simulink model "direct_torque_control"  (Simulink 8.0)
settings: Solver=ode45  StartTime=0.0  StopTime=.4  MaxStep=6e-7  RelTol=1e-3
InitFcn:
  | clear;
  | warning off;
  | wmo=0.0;       %initial speed
  | fso=.996;        %initial stator flux
  | Vdc=700;
  | wo=2*pi*50;
  | 
  | %switching table for DTC
  | a(:,:,1) =[4 0 2;5 7 3];
  | a(:,:,2) =[5 7 6;1 0 2];
  | a(:,:,3) =[1 0 4;3 7 6];
  | a(:,:,4) =[3 7 5;2 0 4];
  | a(:,:,5) =[2 0 1;6 7 5];
  | a(:,:,6) =[6 7 3;4 0 1];
  | clc;
  | %
StopFcn:
  | close all;
  | scrsz = get(0,'ScreenSize');
  | 
  | figure('Name',' Results','OuterPosition',[1 100 scrsz(3)*0.75 scrsz(4)*0.75]);
  | 
  | subplot(1,2,1);
  | plot(fs(:,1),fs(:,2),'-r',fr(:,1),fr(:,2),'-b');
  | axis equal;
  | grid on;
  | title('Flux Spave Vector Trajectory');
  | text(.8,-.85,'rotor flux','color','b');
  | text(-1,-.85,'stator flux','color','r');
  | %figure(2);
  | subplot(1,2,2);
  | plot(an(:,1),unwrap(an(:,2)),'r');
  | grid on;
  | xlabel('Time [s]');
  | ylabel('Rotor flux angle [rad]');
undefined symbols (not defined in the file): a
libraries: simulink x1
settings Model: Creator=Syed Abdul Rahman Kashif  LastModifiedBy=AbdulRahman
settings DataIOCC: SignalLoggingSaveFormat=ModelDataLogs  SignalLoggingName=sigsOut
settings OptimizationCC: BlockReduction=off  BooleanDataType=off
settings DebuggingCC: SaveWithParameterizedLinksMsg=none  SignalResolutionControl=TryResolveAllWithWarning  SolverPrmCheckMsg=none  MultiTaskDSMMsg=warning  MultiTaskCondExecSysMsg=none  FcnCallInpInsideContextMsg=UseLocalSettings  StrictBusMsg=None
settings HardwareCC: TargetUnknown=on
settings RTWCC: IncludeERTFirstTime=on
settings GRTTargetCC: CombineOutputUpdateFcns=off  GRTInterface=on

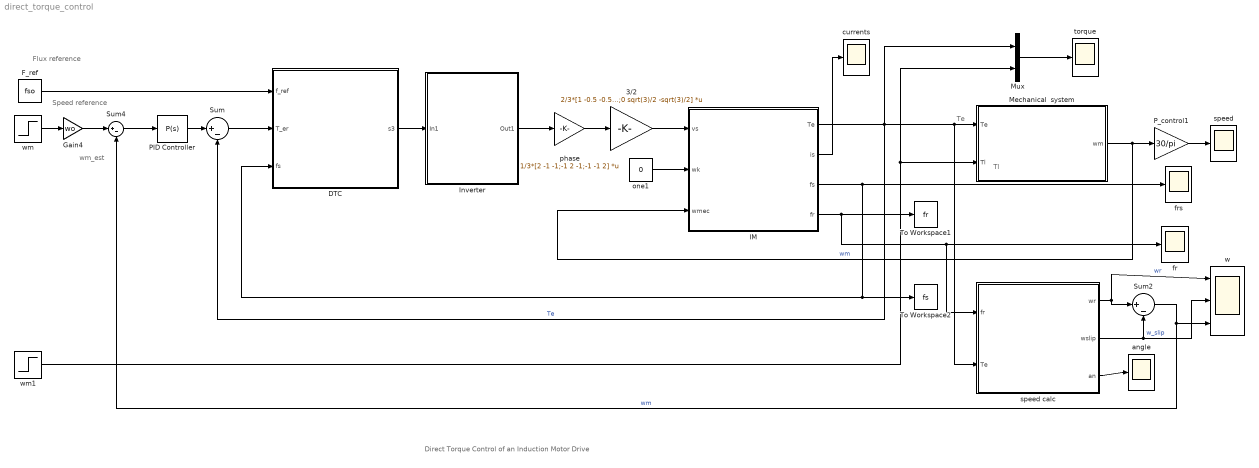
== system direct_torque_control ==
  note: Direct Torque Control of an Induction Motor Drive
  note: Flux reference
  note: Speed reference
  note: Te
  note: Tl
  note: wm_est
  3/2 : Gain  Gain=2/3*[1 -0.5 -0.5;0 sqrt(3)/2 -sqrt(3)/2]  Multiplication=Matrix(K*u)  SaturateOnIntegerOverflow=on  OutDataTypeStr=Inherit: Same as input  ParamDataTypeStr=Inherit: Same as input
  DTC : Subsystem
      mask Display: disp('DTC\ncontroller')
  F_ref : Constant  Value=fso
  Gain4 : Gain  Gain=wo  SaturateOnIntegerOverflow=on  OutDataTypeStr=Inherit: Same as input  ParamDataTypeStr=Inherit: Same as input
  IM : Subsystem  mask{Rs=1.77, Rr=1.34, Lsl=13.93e-3, Lrl=12.12e-3, Lm=369e-3, p=4}
      mask prompts: Rs "Stator resistance [Ohm]"; Rr "Rotor resistance [Ohm]"; Lsl "Stator leakage inductance [H]"; Lrl "Rotor leakage inductance [H]"; Lm "Magnetizing inductance [H]"; p "Number of poles"
      mask Display: disp('INDUCTION\nMOTOR')
  Inverter : Subsystem
  Mechanical  system : Subsystem  mask{J=0.025, Bm=1e-5}
      mask prompts: J "Moment of inertia [Kg.m^2]"; Bm "Torque-speed coefficient"
      mask Display: disp('MECHANICAL\nSYSTEM')
  Mux : Mux  Inputs=2
  PID Controller : simulink/Continuous/PID Controller  Controller=P  TimeDomain=Continuous-time  SampleTime=1  IntegratorMethod=Forward Euler  FilterMethod=Forward Euler  Form=Parallel  P=4  I=1  D=0  N=100  InitialConditionSource=internal  InitialConditionForIntegrator=0  InitialConditionForFilter=0  ExternalReset=none  LimitOutput=on  UpperSaturationLimit=30  LowerSaturationLimit=-30  LinearizeAsGain=on  AntiWindupMode=none  Kb=1  TrackingMode=off  Kt=1  PParamMin=[]  PParamMax=[]  IParamMin=[]  IParamMax=[]  DParamMin=[]  DParamMax=[]  NParamMin=[]  NParamMax=[]  KbParamMin=[]  KbParamMax=[]  KtParamMin=[]  KtParamMax=[]  POutMin=[]  POutMax=[]  IOutMin=[]  IOutMax=[]  DOutMin=[]  DOutMax=[]  NOutMin=[]  NOutMax=[]  KbOutMin=[]  KbOutMax=[]  KtOutMin=[]  KtOutMax=[]  IntegratorOutMin=[]  IntegratorOutMax=[]  FilterOutMin=[]  FilterOutMax=[]  SumOutMin=[]  SumOutMax=[]  SumI1OutMin=[]  SumI1OutMax=[]  SumI2OutMin=[]  SumI2OutMax=[]  SumI3OutMin=[]  SumI3OutMax=[]  SumDOutMin=[]  SumDOutMax=[]  SaturationOutMin=[]  SaturationOutMax=[]  IntegratorContinuousStateAttributes=''  IntegratorStateMustResolveToSignalObject=off  IntegratorRTWStateStorageClass=Auto  FilterContinuousStateAttributes=''  FilterStateMustResolveToSignalObject=off  FilterRTWStateStorageClass=Auto
  P_control1 : Gain  Gain=30/pi  SaturateOnIntegerOverflow=on  OutDataTypeStr=Inherit: Same as input  ParamDataTypeStr=Inherit: Same as input
  Sum : Sum  Inputs=|+-  SaturateOnIntegerOverflow=on
  Sum2 : Sum  Inputs=|+-  SaturateOnIntegerOverflow=on
  Sum4 : Sum  Inputs=|+-  SaturateOnIntegerOverflow=on  InputSameDT=on  OutDataTypeStr=Inherit: Same as first input
  To Workspace1 : ToWorkspace  VariableName=fr  SampleTime=-1
      settings: Decimation=2
  To Workspace2 : ToWorkspace  VariableName=fs  SampleTime=-1
      settings: Decimation=2
  angle : Scope
      settings: TimeRange=0.4  YMin=-3.5  YMax=3.5  SaveName=an  MaxDataPoints=20000  Decimation=20
  currents : Scope
      settings: TimeRange=0.4  YMin=-3.5  YMax=3.5  MaxDataPoints=20000  Decimation=20
  fr : Scope
      settings: TimeRange=1  YMin=-1.5  YMax=1.5  MaxDataPoints=20000  Decimation=20
  frs : Scope
      settings: TimeRange=2  YMin=-1.1  YMax=1.1  SaveName=ScopeData4  MaxDataPoints=20000  Decimation=20
  one1 : Constant  Value=0
  phase : Gain  Gain=1/3*[2 -1 -1;-1 2 -1;-1 -1 2]  Multiplication=Matrix(K*u)  SaturateOnIntegerOverflow=on  OutDataTypeStr=Inherit: Same as input  ParamDataTypeStr=Inherit: Same as input
  speed : Scope
      settings: TimeRange=0.4  YMin=0  YMax=1500  SaveName=ScopeData2  MaxDataPoints=20000  Decimation=20
  speed calc : Subsystem
      mask Display: disp('Speed\nEstimator')
  torque : Scope
      settings: TimeRange=0.4  YMin=-2.5  YMax=32.5  SaveName=ScopeData3  MaxDataPoints=20000  Decimation=20
  w : Scope  NumInputPorts=3
      settings: TimeRange=0.4  YMin=0~-2.5~-50  YMax=350~20~350  SaveName=ScopeData6
  wm : Step  Time=.05  Before=wmo  After=.8  SampleTime=0
  wm1 : Step  Time=.3  After=12  SampleTime=0
  wires:
  F_ref/1 -> DTC/1(f_ref)
  3/2/1 -> IM/1(vs)
  IM/3(fs) -> frs/1, To Workspace2/1, DTC/3(fs)
  one1/1 -> IM/2(wk)
  IM/1(Te) -> Mechanical  system/1(Te), speed calc/2(Te), Sum/2, Mux/1  "Te"
  Mechanical  system/1(wm) -> IM/3(wmec), P_control1/1  "wm"
  IM/2(is) -> currents/1
  wm/1 -> Gain4/1
  Sum/1 -> DTC/2(T_er)
  Mux/1 -> torque/1
  IM/4(fr) -> To Workspace1/1, fr/1, speed calc/1(fr)
  wm1/1 -> Mechanical  system/2(Tl), Mux/2
  speed calc/1(wr) -> Sum2/1, w/1  "wr"
  speed calc/2(wslip) -> w/2, Sum2/2  "w_slip"
  Sum2/1 -> Sum4/2, w/3  "wm"
  phase/1 -> 3/2/1
  Gain4/1 -> Sum4/1
  P_control1/1 -> speed/1
  speed calc/3(an) -> angle/1
  Sum4/1 -> PID Controller/1
  PID Controller/1 -> Sum/1
  DTC/1(s3) -> Inverter/1(In1)
  Inverter/1(Out1) -> phase/1

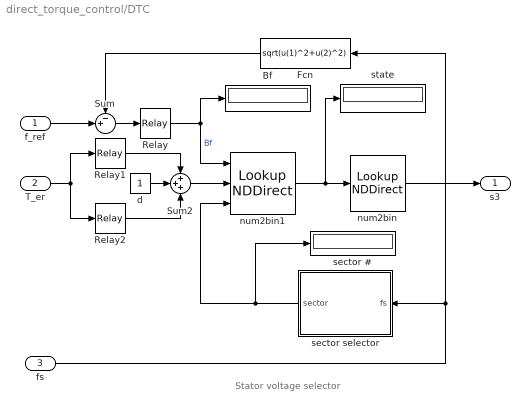
== system direct_torque_control/DTC ==
  note: Stator voltage selector
  f_ref : Inport
  T_er : Inport  Port=2
  fs : Inport  Port=3
  Bf : Display
  Fcn : Fcn  Expr=sqrt(u(1)^2+u(2)^2)
  Relay : Relay  OnSwitchValue=.02  OffSwitchValue=-.02
  Relay1 : Relay  OnSwitchValue=.2  OffSwitchValue=0  ZeroCross=off
  Relay2 : Relay  OnSwitchValue=0  OffSwitchValue=-.2  OnOutputValue=0  OffOutputValue=-1  ZeroCross=off
  Sum : Sum  Inputs=-+|  SaturateOnIntegerOverflow=on  InputSameDT=on  OutDataTypeStr=Inherit: Same as first input
  Sum2 : Sum  Inputs=+++  SaturateOnIntegerOverflow=on  InputSameDT=on  OutDataTypeStr=Inherit: Same as first input
  d : Constant
  num2bin : LookupNDDirect  InputsSelectThisObjectFromTable=Column  Table=[0 0 0;1 0 0;0 1 0;1 1 0;0 0 1;1 0 1;0 1 1;1 1 1]'  DiagnosticForOutOfRangeInput=Error
  num2bin1 : LookupNDDirect  NumberOfTableDimensions=3  Table=a  DiagnosticForOutOfRangeInput=Error
  sector # : Display
  sector selector : Subsystem
  state : Display
  s3 : Outport
  wires:
  num2bin1/1 -> state/1, num2bin/1
  Sum/1 -> Relay/1
  Relay/1 -> Bf/1, num2bin1/1  "Bf"
  Fcn/1 -> Sum/1
  Sum2/1 -> num2bin1/2
  Relay1/1 -> Sum2/1
  Relay2/1 -> Sum2/3
  d/1 -> Sum2/2
  T_er/1 -> Relay2/1, Relay1/1
  f_ref/1 -> Sum/2
  num2bin/1 -> s3/1
  fs/1 -> Fcn/1, sector selector/1(fs)
  sector selector/1(sector) -> num2bin1/3, sector #/1

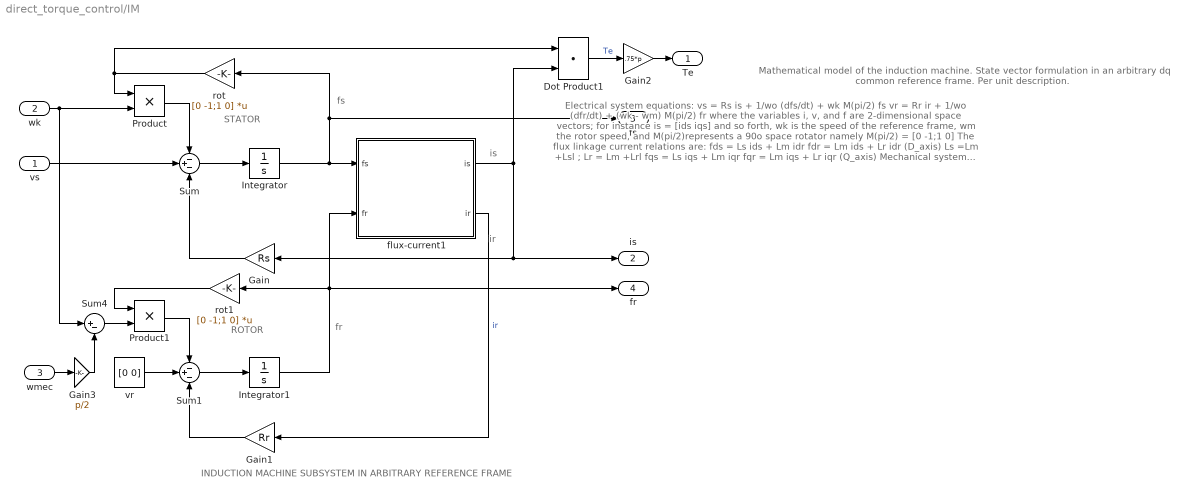
== system direct_torque_control/IM ==
  note: ROTOR
  note: STATOR
  note: fs
  note: fr
  note: is
  note: INDUCTION MACHINE SUBSYSTEM IN ARBITRARY REFERENCE FRAME
  note: ir
  note: Mathematical model of the induction machine.
      | State vector formulation in an arbitrary dq common reference frame.
      | Per unit description.
  note: Electrical  system equations:
      |             vs = Rs is + 1/wo (dfs/dt) + wk M(pi/2) fs
      |             vr  = Rr ir  + 1/wo (dfr/dt)  + (wk - wm) M(pi/2) fr
      |       where the variables i, v, and f are 2-dimensional space vectors; for instance
      |             is = [ids iqs] and so forth,
      |       wk is the speed of the reference frame, wm the rotor speed,
      |       and M(pi/2)represents a 90o space rotator namely M(pi/2) = [0 -1;1 0]
      |
      |     The flux linkage current relations are:
      |           fds = Ls ids + Lm idr
      |           fdr =  Lm ids + Lr idr          (D_axis)
      |                                                                        Ls =Lm +Lsl  ; Lr = Lm +Lrl
      |           fqs = Ls iqs + Lm iqr
      |           fqr  = Lm iqs + Lr iqr         (Q_axis)
      |
      |  Mechanical system equations:
      |              Te = 2H (dwm/dt ) + Bm wm + Tl
      |             where Te = fs (cross) is = M(pi/2) fs (dot) is = fds iqs - fqs ids
      |                               = fs x is = M(pi/2) fs . is
      |                               = ir x fr   = Lm (ir x is) = Lm/Lr (fr x is)
      |                               = 1/Lm' (fr x fs)        Lm' =Lm c/(1-c)   c = 1 - Lm^2/(Ls Lr)
  vs : Inport
  wk : Inport  Port=2
  wmec : Inport  Port=3
  Dot Product1 : DotProduct  InputSameDT=on  OutDataTypeStr=Inherit: Inherit via internal rule
  Gain : Gain  Gain=Rs  SaturateOnIntegerOverflow=on  OutDataTypeStr=Inherit: Same as input  ParamDataTypeStr=Inherit: Same as input
  Gain1 : Gain  Gain=Rr  SaturateOnIntegerOverflow=on  OutDataTypeStr=Inherit: Same as input  ParamDataTypeStr=Inherit: Same as input
  Gain2 : Gain  Gain=.75*p  SaturateOnIntegerOverflow=on  OutDataTypeStr=Inherit: Same as input  ParamDataTypeStr=Inherit: Same as input
  Gain3 : Gain  Gain=p/2  SaturateOnIntegerOverflow=on  OutDataTypeStr=Inherit: Same as input  ParamDataTypeStr=Inherit: Same as input
  Integrator : Integrator  InitialCondition=[fso 0]
  Integrator1 : Integrator  InitialCondition=[fso 0]
  Product : Product  SaturateOnIntegerOverflow=on  InputSameDT=on  OutDataTypeStr=Inherit: Same as first input
  Product1 : Product  SaturateOnIntegerOverflow=on  InputSameDT=on  OutDataTypeStr=Inherit: Same as first input
  Sum : Sum  Inputs=-+-  SaturateOnIntegerOverflow=on  InputSameDT=on  OutDataTypeStr=Inherit: Same as first input
  Sum1 : Sum  Inputs=-+-  SaturateOnIntegerOverflow=on  InputSameDT=on  OutDataTypeStr=Inherit: Same as first input
  Sum4 : Sum  Inputs=|+-  SaturateOnIntegerOverflow=on  InputSameDT=on  OutDataTypeStr=Inherit: Same as first input
  flux-current1 : Subsystem
      mask Display: disp('FLUX-CURRENT\nRELATIONS')
  rot : Gain  Gain=[0 -1;1 0]  Multiplication=Matrix(K*u)  SaturateOnIntegerOverflow=on  OutDataTypeStr=Inherit: Same as input  ParamDataTypeStr=Inherit: Same as input
  rot1 : Gain  Gain=[0 -1;1 0]  Multiplication=Matrix(K*u)  SaturateOnIntegerOverflow=on  OutDataTypeStr=Inherit: Same as input  ParamDataTypeStr=Inherit: Same as input
  vr : Constant  Value=[0 0]
  Te : Outport
  is : Outport  Port=2
  fs : Outport  Port=3
  fr : Outport  Port=4
  wires:
  Gain/1 -> Sum/3
  vr/1 -> Sum1/2
  Gain1/1 -> Sum1/3
  flux-current1/2(ir) -> Gain1/1  "ir"
  Integrator/1 -> flux-current1/1(fs), rot/1, fs/1
  Integrator1/1 -> flux-current1/2(fr), rot1/1, fr/1
  Product1/1 -> Sum1/1
  rot1/1 -> Product1/1
  Product/1 -> Sum/1
  rot/1 -> Product/1, Dot Product1/1
  Sum4/1 -> Product1/2
  Sum/1 -> Integrator/1
  Sum1/1 -> Integrator1/1
  flux-current1/1(is) -> Gain/1, is/1, Dot Product1/2
  Dot Product1/1 -> Gain2/1  "Te"
  vs/1 -> Sum/2
  wk/1 -> Product/2, Sum4/1
  wmec/1 -> Gain3/1
  Gain2/1 -> Te/1
  Gain3/1 -> Sum4/2

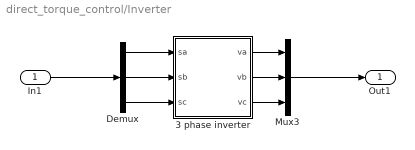
== system direct_torque_control/Inverter ==
  In1 : Inport
  3 phase inverter : Subsystem
  Demux : Demux  Outputs=3
  Mux3 : Mux  Inputs=3
  Out1 : Outport
  wires:
  In1/1 -> Demux/1
  3 phase inverter/3(vc) -> Mux3/3
  3 phase inverter/2(vb) -> Mux3/2
  3 phase inverter/1(va) -> Mux3/1
  Demux/3 -> 3 phase inverter/3(sc)
  Demux/2 -> 3 phase inverter/2(sb)
  Demux/1 -> 3 phase inverter/1(sa)
  Mux3/1 -> Out1/1

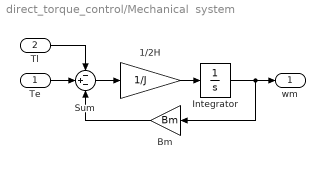
== system direct_torque_control/Mechanical  system ==
  Te : Inport
  Tl : Inport  Port=2
  1/2H : Gain  Gain=1/J  SaturateOnIntegerOverflow=on  OutDataTypeStr=Inherit: Same as input  ParamDataTypeStr=Inherit: Same as input
  Bm : Gain  Gain=Bm  SaturateOnIntegerOverflow=on  OutDataTypeStr=Inherit: Same as input  ParamDataTypeStr=Inherit: Same as input
  Integrator : Integrator  InitialCondition=wmo
  Sum : Sum  Inputs=-+-  SaturateOnIntegerOverflow=on  InputSameDT=on  OutDataTypeStr=Inherit: Same as first input
  wm : Outport
  wires:
  Tl/1 -> Sum/1
  Te/1 -> Sum/2
  Integrator/1 -> wm/1, Bm/1
  Bm/1 -> Sum/3
  Sum/1 -> 1/2H/1
  1/2H/1 -> Integrator/1

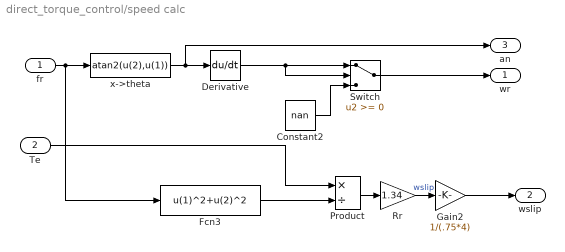
== system direct_torque_control/speed calc ==
  fr : Inport
  Te : Inport  Port=2
  Constant2 : Constant  Value=nan
  Derivative : Derivative
  Fcn3 : Fcn  Expr=u(1)^2+u(2)^2
  Gain2 : Gain  Gain=1/(.75*4)  SaturateOnIntegerOverflow=on  OutDataTypeStr=Inherit: Same as input  ParamDataTypeStr=Inherit: Same as input
  Product : Product  Inputs=*/  SaturateOnIntegerOverflow=on  InputSameDT=on  OutDataTypeStr=Inherit: Same as first input
  Rr : Gain  Gain=1.34  SaturateOnIntegerOverflow=on  OutDataTypeStr=Inherit: Same as input  ParamDataTypeStr=Inherit: Same as input
  Switch : Switch  ZeroCross=off  SaturateOnIntegerOverflow=on
  x->theta : Fcn  Expr=atan2(u(2),u(1))
  wr : Outport
  wslip : Outport  Port=2
  an : Outport  Port=3
  wires:
  Switch/1 -> wr/1
  Constant2/1 -> Switch/3
  Derivative/1 -> Switch/1, Switch/2
  fr/1 -> x->theta/1, Fcn3/1
  x->theta/1 -> Derivative/1, an/1
  Fcn3/1 -> Product/2
  Product/1 -> Rr/1
  Te/1 -> Product/1
  Rr/1 -> Gain2/1  "wslip"
  Gain2/1 -> wslip/1

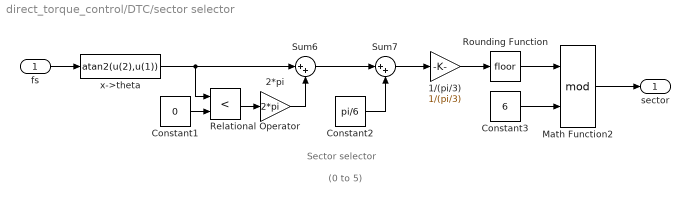
== system direct_torque_control/DTC/sector selector ==
  note: Sector selector
  note: (0 to 5)
  fs : Inport
  1/(pi/3) : Gain  Gain=1/(pi/3)  SaturateOnIntegerOverflow=on  OutDataTypeStr=Inherit: Same as input  ParamDataTypeStr=Inherit: Same as input
  2*pi : Gain  Gain=2*pi  SaturateOnIntegerOverflow=on  OutDataTypeStr=Inherit: Same as input  ParamDataTypeStr=Inherit: Same as input
  Constant1 : Constant  Value=0
  Constant2 : Constant  Value=pi/6
  Constant3 : Constant  Value=6
  Math Function2 : Math  Operator=mod  SaturateOnIntegerOverflow=on
  Relational Operator : RelationalOperator  Operator=<  InputSameDT=on
  Rounding Function : Rounding
  Sum6 : Sum  Inputs=|++  SaturateOnIntegerOverflow=on  InputSameDT=on  OutDataTypeStr=Inherit: Same as first input
  Sum7 : Sum  Inputs=|++  SaturateOnIntegerOverflow=on  InputSameDT=on  OutDataTypeStr=Inherit: Same as first input
  x->theta : Fcn  Expr=atan2(u(2),u(1))
  sector : Outport
  wires:
  Constant1/1 -> Relational Operator/2
  Relational Operator/1 -> 2*pi/1
  2*pi/1 -> Sum6/2
  Sum6/1 -> Sum7/1
  Constant2/1 -> Sum7/2
  Sum7/1 -> 1/(pi/3)/1
  1/(pi/3)/1 -> Rounding Function/1
  Rounding Function/1 -> Math Function2/1
  Constant3/1 -> Math Function2/2
  fs/1 -> x->theta/1
  Math Function2/1 -> sector/1
  x->theta/1 -> Relational Operator/1, Sum6/1

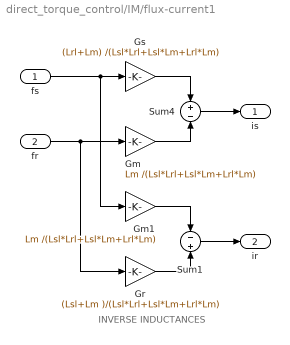
== system direct_torque_control/IM/flux-current1 ==
  note: INVERSE INDUCTANCES
  fs : Inport
  fr : Inport  Port=2
  Gm : Gain  Gain=Lm /(Lsl*Lrl+Lsl*Lm+Lrl*Lm)  SaturateOnIntegerOverflow=on  OutDataTypeStr=Inherit: Same as input  ParamDataTypeStr=Inherit: Same as input
  Gm1 : Gain  Gain=Lm /(Lsl*Lrl+Lsl*Lm+Lrl*Lm)  SaturateOnIntegerOverflow=on  OutDataTypeStr=Inherit: Same as input  ParamDataTypeStr=Inherit: Same as input
  Gr : Gain  Gain=(Lsl+Lm )/(Lsl*Lrl+Lsl*Lm+Lrl*Lm)  SaturateOnIntegerOverflow=on  OutDataTypeStr=Inherit: Same as input  ParamDataTypeStr=Inherit: Same as input
  Gs : Gain  Gain=(Lrl+Lm) /(Lsl*Lrl+Lsl*Lm+Lrl*Lm)  SaturateOnIntegerOverflow=on  OutDataTypeStr=Inherit: Same as input  ParamDataTypeStr=Inherit: Same as input
  Sum1 : Sum  Inputs=-+  SaturateOnIntegerOverflow=on  InputSameDT=on  OutDataTypeStr=Inherit: Same as first input
  Sum4 : Sum  Inputs=+-  SaturateOnIntegerOverflow=on  InputSameDT=on  OutDataTypeStr=Inherit: Same as first input
  is : Outport
  ir : Outport  Port=2
  wires:
  fs/1 -> Gs/1, Gm1/1
  Gs/1 -> Sum4/1
  fr/1 -> Gm/1, Gr/1
  Gm/1 -> Sum4/2
  Sum4/1 -> is/1
  Gm1/1 -> Sum1/1
  Gr/1 -> Sum1/2
  Sum1/1 -> ir/1

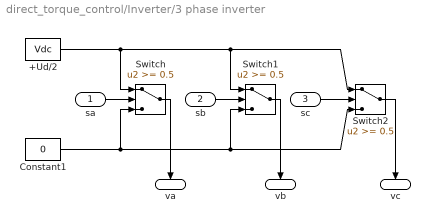
== system direct_torque_control/Inverter/3 phase inverter ==
  sa : Inport
  sb : Inport  Port=2
  sc : Inport  Port=3
  +Ud/2 : Constant  Value=Vdc
  Constant1 : Constant  Value=0
  Switch : Switch  Threshold=0.5  SaturateOnIntegerOverflow=on  InputSameDT=on
  Switch1 : Switch  Threshold=0.5  SaturateOnIntegerOverflow=on  InputSameDT=on
  Switch2 : Switch  Threshold=0.5  SaturateOnIntegerOverflow=on  InputSameDT=on
  va : Outport  InitialOutput=0
  vb : Outport  Port=2  InitialOutput=0
  vc : Outport  Port=3  InitialOutput=0
  wires:
  Switch1/1 -> vb/1
  Switch2/1 -> vc/1
  sc/1 -> Switch2/2
  sb/1 -> Switch1/2
  Switch/1 -> va/1
  sa/1 -> Switch/2
  Constant1/1 -> Switch2/3, Switch1/3, Switch/3
  +Ud/2/1 -> Switch2/1, Switch1/1, Switch/1
